simulink model "q3_model"  (R2018a)
settings: Solver=VariableStepAuto  StartTime=0.0  StopTime=t_f  FixedStep=1  RelTol=1e-7  AbsTol=1e-7
values from neighbouring files (symbols this model uses):
  c = 0.1    [q3.m]
  I_b = [100 1 2; 1 150 3; 2 3 200]    [q1.m]    (also in q3.m)
  I_d = 1    [q3.m]
  m_N_t0 = 7.76*[sqrt(2)/2 sqrt(2)/2 0].'    [q3.m]
  omega_b_t0 = [0.02 0 0.2].'    [q3.m]
  q_t0 = [0 0 0 1].'    [q1.m]    (also in q3.m)
  shat_N = [0 0 1].'    [q3.m]
libraries: sharedtransform x2, vrlib x1
settings Model: Creator=Padraig Lysandrou  LastModifiedBy=Padraig Lysandrou

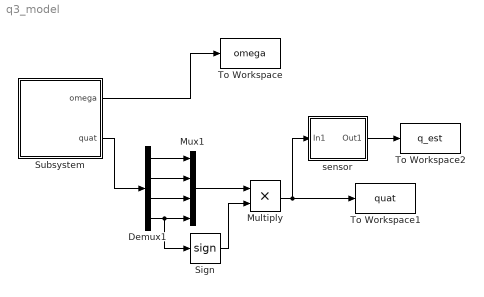
== system q3_model ==
  Demux1 : Demux
  Multiply : Product
  Mux1 : Mux
  Sign : Signum
  Subsystem : Subsystem
  To Workspace : ToWorkspace  VariableName=omega  SaveFormat=Timeseries  SampleTime=-1
  To Workspace1 : ToWorkspace  VariableName=quat  SaveFormat=Timeseries  SampleTime=-1
  To Workspace2 : ToWorkspace  VariableName=q_est  SaveFormat=Timeseries  SampleTime=-1
  sensor : Subsystem
  wires:
  Subsystem/1("omega ") -> To Workspace/1
  sensor/1(Out1) -> To Workspace2/1
  Subsystem/2(quat) -> Demux1/1
  Demux1/1 -> Mux1/1
  Demux1/2 -> Mux1/2
  Demux1/3 -> Mux1/3
  Demux1/4 -> Sign/1, Mux1/4
  Sign/1 -> Multiply/2
  Mux1/1 -> Multiply/1
  Multiply/1 -> sensor/1(In1), To Workspace1/1

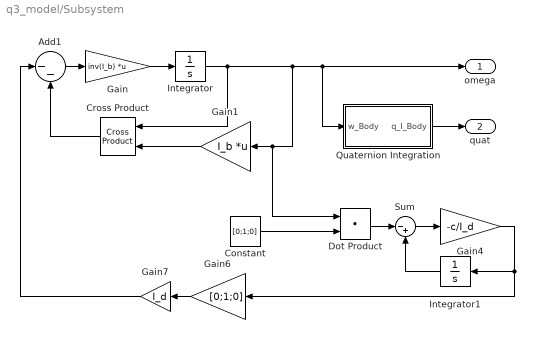
== system q3_model/Subsystem ==
  Add1 : Sum  Inputs=|--
  Constant : Constant  Value=[0;1;0]
  Cross Product : vrlib/Utilities/Cross Product
      settings: SourceProductBaseCode=VR
  Dot Product : DotProduct  InputSameDT=on  OutDataTypeStr=Inherit: Inherit via internal rule
  Gain : Gain  Gain=inv(I_b)  Multiplication=Matrix(K*u) (u vector)
  Gain1 : Gain  Gain=I_b  Multiplication=Matrix(K*u) (u vector)
  Gain4 : Gain  Gain=-c/I_d
  Gain6 : Gain  Gain=[0;1;0]
  Gain7 : Gain  Gain=I_d
  Integrator : Integrator  InitialCondition=omega_b_t0
  Integrator1 : Integrator
  Quaternion Integration : Subsystem
  Sum : Sum  Inputs=|-+
  "omega " : Outport
  quat : Outport  Port=2
  wires:
  Integrator/1 -> Quaternion Integration/1(w_Body), "omega "/1, Gain1/1, Dot Product/1, Cross Product/1
  Gain/1 -> Integrator/1
  Gain1/1 -> Cross Product/2
  Add1/1 -> Gain/1
  Quaternion Integration/1(q_I_Body) -> quat/1
  Cross Product/1 -> Add1/2
  Integrator1/1 -> Sum/2
  Sum/1 -> Gain4/1
  Gain4/1 -> Integrator1/1, Gain6/1
  Dot Product/1 -> Sum/1
  Constant/1 -> Dot Product/2
  Gain7/1 -> Add1/1
  Gain6/1 -> Gain7/1

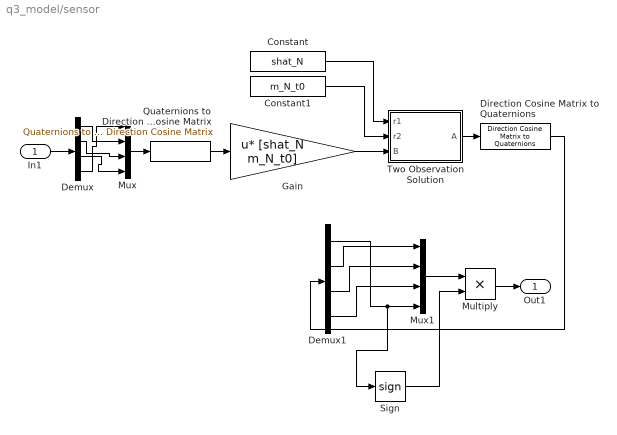
== system q3_model/sensor ==
  In1 : Inport
  Constant : Constant  Value=shat_N
  Constant1 : Constant  Value=m_N_t0
  Demux : Demux
  Demux1 : Demux
  Direction Cosine Matrix to Quaternions : sharedtransform/Direction Cosine Matrix  to Quaternions  aMode=0  action=None  tolerance=eps(2)
      settings: SourceProductName=Aerospace Blockset  SourceProductBaseCode=AE
  Gain : Gain  Gain=[shat_N m_N_t0]  Multiplication=Matrix(u*K)
  Multiply : Product
  Mux : Mux
  Mux1 : Mux
  Quaternions to Direction Cosine Matrix : sharedtransform/Quaternions to  Direction Cosine Matrix  aMode=aMode
      settings: SourceProductName=Aerospace Blockset  SourceProductBaseCode=AE
  Sign : Signum
  "Two Observation Solution " : MATLAB Function  TreatAsAtomicUnit=on
  Out1 : Outport
  wires:
  Demux/1 -> Mux/2
  Demux/2 -> Mux/3
  Demux/3 -> Mux/4
  Mux/1 -> Quaternions to Direction Cosine Matrix/1
  Demux/4 -> Mux/1
  In1/1 -> Demux/1
  Quaternions to Direction Cosine Matrix/1 -> Gain/1
  Gain/1 -> "Two Observation Solution "/3(B)
  Constant/1 -> "Two Observation Solution "/1(r1)
  Constant1/1 -> "Two Observation Solution "/2(r2)
  "Two Observation Solution "/1(A) -> Direction Cosine Matrix to Quaternions/1
  Direction Cosine Matrix to Quaternions/1 -> Demux1/1
  Demux1/1 -> Sign/1, Mux1/4
  Demux1/2 -> Mux1/1
  Demux1/3 -> Mux1/2
  Demux1/4 -> Mux1/3
  Sign/1 -> Multiply/2
  Mux1/1 -> Multiply/1
  Multiply/1 -> Out1/1

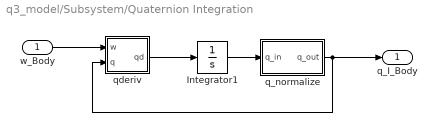
== system q3_model/Subsystem/Quaternion Integration ==
  w_Body : Inport
  Integrator1 : Integrator  InitialCondition=q_t0
  q_normalize : Subsystem
  qderiv : Subsystem
  q_I_Body : Outport
  wires:
  w_Body/1 -> qderiv/1(w)
  q_normalize/1(q_out) -> qderiv/2(q), q_I_Body/1
  Integrator1/1 -> q_normalize/1(q_in)
  qderiv/1(qd) -> Integrator1/1

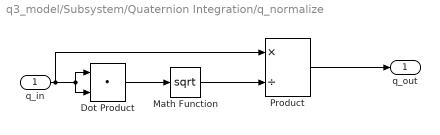
== system q3_model/Subsystem/Quaternion Integration/q_normalize ==
  q_in : Inport  PortDimensions=4
  Dot Product : DotProduct  InputSameDT=on  OutDataTypeStr=Inherit: Inherit via internal rule
  Math Function : Math  Operator=sqrt  SaturateOnIntegerOverflow=on
  Product : Product  Inputs=*/  SaturateOnIntegerOverflow=on  InputSameDT=on  OutDataTypeStr=Inherit: Same as first input
  q_out : Outport
  wires:
  Product/1 -> q_out/1
  Math Function/1 -> Product/2
  Dot Product/1 -> Math Function/1
  q_in/1 -> Dot Product/2, Dot Product/1, Product/1

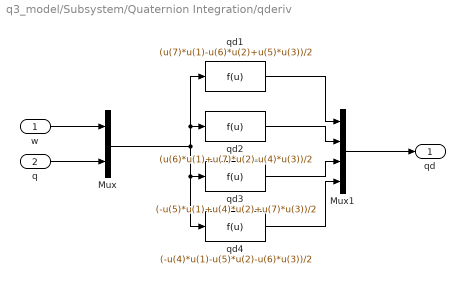
== system q3_model/Subsystem/Quaternion Integration/qderiv ==
  w : Inport
  q : Inport  Port=2
  Mux : Mux  Inputs=2
  Mux1 : Mux
  qd1 : Fcn  Expr=(u(7)*u(1)-u(6)*u(2)+u(5)*u(3))/2
  qd2 : Fcn  Expr=(u(6)*u(1)+u(7)*u(2)-u(4)*u(3))/2
  qd3 : Fcn  Expr=(-u(5)*u(1)+u(4)*u(2)+u(7)*u(3))/2
  qd4 : Fcn  Expr=(-u(4)*u(1)-u(5)*u(2)-u(6)*u(3))/2
  qd : Outport
  wires:
  Mux1/1 -> qd/1
  qd4/1 -> Mux1/4
  qd3/1 -> Mux1/3
  qd2/1 -> Mux1/2
  qd1/1 -> Mux1/1
  Mux/1 -> qd4/1, qd3/1, qd2/1, qd1/1
  q/1 -> Mux/2
  w/1 -> Mux/1

== matlab function q3_model/sensor/Two Observation Solution  ==
  data: r1 input; r2 input; B input; A output
function A = twoobs(r1, r2, B)
lmax = 0;
bx = zeros(3,1);
rx = zeros(3,1);
A = zeros(3,3);
q_out = zeros(4,1);

a1 = 0.95;
a2 = 0.05;
b1 = B(:,1);
b2 = B(:,2)+0.1;
l0 = a1+a2;
lmax = (a1^2 + a2^2 + 2*a1*a2*(dot(b1,b2)*dot(r1,r2) ...
    + (norm(crs(b1)*b2)*norm(crs(r1)*r2))))^(0.5);
bx = (crs(b1)*b2)/norm(crs(b1)*b2);
rx = (crs(r1)*r2)/norm(crs(r1)*r2);
A = (a1/lmax)*(b1*r1.' + (crs(b1)*bx)*((crs(r1)*rx).')) + ...
    (a2/lmax)*(b2*r2.' + (crs(b2)*bx)*((crs(r2)*rx).')) + bx*rx.';
% A = A.';
end
